simulink model "hotelsamofuzzy2012B"  (R2012b)
settings: Solver=ode45  StartTime=0.0  StopTime=1  RelTol=1e-3
libraries: fuzblock x1
settings Model: Creator=korisnik  LastModifiedBy=Aldin
settings DebuggingCC: FrameProcessingCompatibilityMsg=error
settings CodeAppCC: CustomSymbolStrType=$N$R$M_T
settings GRTTargetCC: CodeReplacementLibrary=C89/C90 (ANSI)

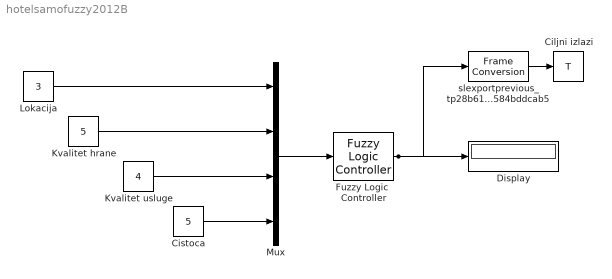
== system hotelsamofuzzy2012B ==
  Ciljni izlazi : ToWorkspace  VariableName=T  SampleTime=-1
  Cistoca : Constant  Value=5
  Display : Display
  Fuzzy Logic  Controller : fuzblock/Fuzzy Logic  Controller  FIS=restoran
  Kvalitet hrane : Constant  Value=5
  Kvalitet usluge : Constant  Value=4
  Lokacija : Constant  Value=3
  Mux : Mux
  slexportprevious_tp28b61391_ad36_42bf_ace4_1c584bddcab5 : FrameConversion  OutFrame=Sample-based
  wires:
  Lokacija/1 -> Mux/1
  Mux/1 -> Fuzzy Logic  Controller/1
  Fuzzy Logic  Controller/1 -> Display/1, slexportprevious_tp28b61391_ad36_42bf_ace4_1c584bddcab5/1
  Kvalitet usluge/1 -> Mux/3
  Cistoca/1 -> Mux/4
  Kvalitet hrane/1 -> Mux/2
  slexportprevious_tp28b61391_ad36_42bf_ace4_1c584bddcab5/1 -> Ciljni izlazi/1
